simulink model "suspension_system"  (R2020b)
settings: Solver=VariableStepAuto  StartTime=0.0  StopTime=100  RelTol=1e-3
model workspace (MAT data in the model file):
  b = 1000
  k1 = 25000
  m1 = 500
settings Model: Creator=Administrator  LastModifiedBy=Administrator

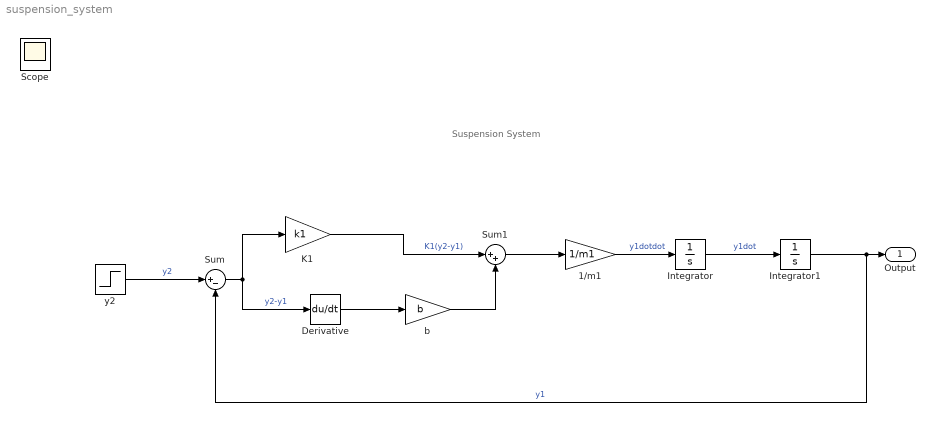
== system suspension_system ==
  note: Suspension System
  1/m1 : Gain  Gain=1/m1
  Derivative : Derivative
  Integrator : Integrator
  Integrator1 : Integrator
  K1 : Gain  Gain=k1
  Sum : Sum  Inputs=|+-
  Sum1 : Sum  Inputs=|++
  b : Gain  Gain=b
  y2 : Step  SampleTime=0
  Output : Outport
  Scope : Scope
  wires:
  y2/1 -> Sum/1  "y2"
  Sum/1 -> Derivative/1, K1/1  "y2-y1"
  K1/1 -> Sum1/1  "K1(y2-y1)"
  Derivative/1 -> b/1
  b/1 -> Sum1/2
  Sum1/1 -> 1/m1/1
  1/m1/1 -> Integrator/1  "y1dotdot"
  Integrator/1 -> Integrator1/1  "y1dot"
  Integrator1/1 -> Output/1, Sum/2  "y1"
